simulink model "sampleModel1395_1_sub_sub_sub"  (R2023a)
settings: Solver=VariableStepAuto  StartTime=0.0  StopTime=10.0  RelTol=1e-3
libraries: simulink x1, hdlsllib x1
settings Model: Creator=user1  LastModifiedBy=user1

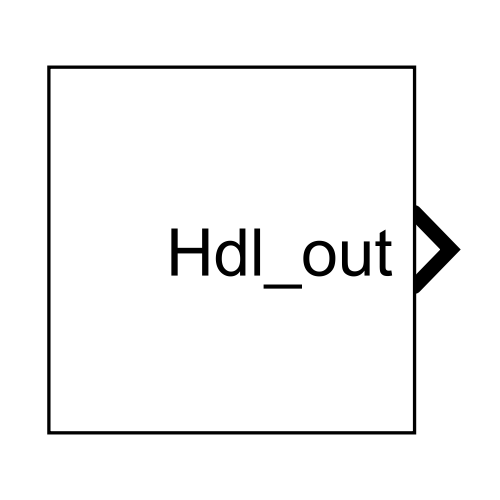
[thumbnail: Simulink's stored preview of the top-level diagram]
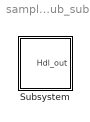
== system sampleModel1395_1_sub_sub_sub ==
  Subsystem : Subsystem

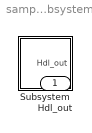
== system sampleModel1395_1_sub_sub_sub/Subsystem ==
  Subsystem : Subsystem
  Hdl_out : Outport  OutDataTypeStr=uint8

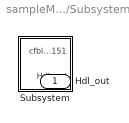
== system sampleModel1395_1_sub_sub_sub/Subsystem/Subsystem ==
  Subsystem : Subsystem
  Hdl_out : Outport  OutDataTypeStr=uint8

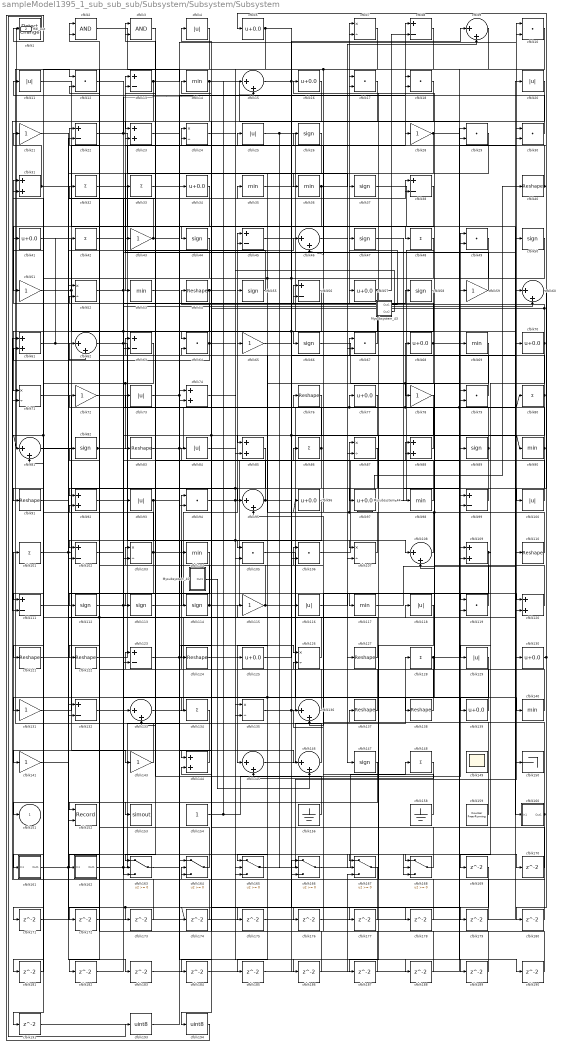
== system sampleModel1395_1_sub_sub_sub/Subsystem/Subsystem/Subsystem ==
  Mysubsystem_40 : Subsystem  TreatAsAtomicUnit=on  RTWFcnName=Mysubsystem_40
      settings: RTWFcnNameOpts=User specified  RTWFileNameOpts=Use function name
  Mysubsystem_43 : Subsystem  TreatAsAtomicUnit=on  RTWFcnName=Mysubsystem_43
      settings: RTWFcnNameOpts=User specified  RTWFileNameOpts=Use function name
  Mysubsystem_44 : Subsystem  TreatAsAtomicUnit=on  RTWFcnName=Mysubsystem_44
      settings: RTWFcnNameOpts=User specified  RTWFileNameOpts=Use function name
  cfblk1 : simulink/Logic and Bit Operations/Detect Change  vinit=0  OutDataTypeStr=uint8
      settings: LibrarySourceBlock=|
      | hdlsllib/Logic and Bit
      | Operations/Detect
      | Change
  cfblk{10,12,17..18,29..30,49,64,67,79,94,105..106,119} (14 alike) : DotProduct  OutDataTypeStr=uint8
  cfblk{4,11,20,25,73,84,93,100,116,118,129} (11 alike) : Abs  OutDataTypeStr=uint8  SaturateOnIntegerOverflow=off
  cfblk{32..33,42,48,80,86,101,128,134,148} (10 alike) : Sum  Inputs=+  OutDataTypeStr=uint8
  cfblk{8,13,22,38,45,56,63,99,102,111,123,132} (12 alike) : Sum  Inputs=+-  OutDataTypeStr=uint8
  cfblk{7,24,52,71,87,103,107,126,135} (9 alike) : Product  Inputs=*/  OutDataTypeStr=uint8  RndMeth=Zero  SaturateOnIntegerOverflow=on
  cfblk{14,35..36,53,69,90,98,104,117,140} (10 alike) : MinMax  OutDataTypeStr=uint8
  cfblk{9,15,46,60,62,81,95,108,133,136,145..146} (12 alike) : Sum  Inputs=|++  OutDataTypeStr=uint8
  cfblk{23,31,61,74,85,88,92,109,120,144} (10 alike) : Sum  OutDataTypeStr=uint8
  cfblk{40,54,76,83,91,110,121..122,124,127,137..138} (12 alike) : Reshape
  cfblk{26,37,44,47,50,55,58,66,82,89,112..114,147} (14 alike) : Signum
  cfblk{21,28,43,51,59,65,72,78,115,131,141,143} (12 alike) : Gain  OutDataTypeStr=uint8
  cfblk{5,16,34,41,57,68,70,77,96..97,125,130,139} (13 alike) : Bias  Bias=0.0  SaturateOnIntegerOverflow=off
  cfblk149 : Scope
      settings: Floating=on
  cfblk150 : Terminator
  cfblk152 : Record  FileSettingsInternal="{\"entries\":[{\"content\":{\"excelSettings\":{\"content\":{},\"type\":\"Streamout.ExcelSettings\"}},\"type\":\"Streamout.FileSettingStorage\",\"uuid\":\"\"}],\"packageUris\":[\"http:\\/\\/schema.mathworks.com\\/mf0\\/streamout_blocks\\/R2020a\"],\"version\":\"1.0\"}"  Layout=[1 1]  SignalsInternal="{\"entries\":[{\"content\":{\"signals\":[{\"content\":{\"blockPath\":[],\"dimensions\":[1],\"domain\":\"\",\"lineColor\":\"#a2142f\",\"plots\":[1],\"port\":1,\"signalID\":10034,\"signalName\":\"cfblk128\"},\"type\":\"RecordBlkView.Signal\",\"uuid\":\"\"},{\"content\":{\"blockPath\":[],\"dimensions\":[1],\"domain\":\"\",\"lineColor\":\"#139fff\",\"plots\":[1],\"port\":2,\"signalID\":10037,\"signalName\":\"cfblk26\"},\"type\":\"RecordBlkView.Signal\",\"uuid\":\"\"}]},\"type\":\"RecordBlkView.InputSignals\",\"uuid\":\"\"}],\"packageUris\":[\"http:\\/\\/schema.mathworks.com\\/mf0\\/streamout_blocks\\/R2020a\"],\"version\":\"1.0\"}"  VisualizationBindings="{\"xyplotplugin\":{\"info\":[{\"series\":[{\"bindingParametersList\":[{\"parameter\":\"X-Axis\",\"signalID\":10034,\"signalName\":\"cfblk128\"},{\"parameter\":\"Y-Axis\",\"signalID\":10037,\"signalName\":\"cfblk26\"}],\"seriesID\":30832}],\"subplotID\":1}]}}"  CompatibilityTag=XY  st=-1
  cfblk153 : ToWorkspace  VariableName=simout  SaveFormat=Timeseries  SampleTime=-1
  cfblk154 : Constant  OutDataTypeStr=uint8  SampleTime=-1
  cfblk156 : Ground
  cfblk158 : Ground
  cfblk159 : hdlsllib/Sources/Counter Free-Running  NumBits=16  tsamp=-1
  cfblk160 : Subsystem
      settings: LibrarySourceBlock=|
      | hdlsllib/Ports &
      | Subsystems/Subsystem
  cfblk161 : Subsystem
      settings: LibrarySourceBlock=|
      | hdlsllib/Ports &
      | Subsystems/Subsystem
  cfblk162 : Subsystem
      settings: LibrarySourceBlock=|
      | hdlsllib/Ports &
      | Subsystems/Subsystem
  cfblk{163..168} (6 alike) : Switch  OutDataTypeStr=uint8  SaturateOnIntegerOverflow=off  InputSameDT=off
  cfblk{169..191} (23 alike) : Delay  SampleTime=1
  cfblk193 : DataTypeConversion  OutDataTypeStr=uint8  SaturateOnIntegerOverflow=off  RndMeth=Floor
  cfblk194 : DataTypeConversion  OutDataTypeStr=uint8  SaturateOnIntegerOverflow=off  RndMeth=Floor
  cfblk2 : Logic  AllPortsSameDT=off  OutDataTypeStr=boolean
  cfblk3 : Logic  AllPortsSameDT=off  OutDataTypeStr=boolean
  cfblk151 : Outport  OutDataTypeStr=uint8  VectorParamsAs1DForOutWhenUnconnected=off
  Hdl_out : Outport  Port=2  OutDataTypeStr=uint8
  wires:
  cfblk92/1 -> cfblk108/1
  cfblk154/1 -> cfblk15/1, cfblk49/1
  cfblk165/1 -> cfblk10/1
  cfblk11/1 -> cfblk48/1
  cfblk112/1 -> cfblk88/2, cfblk117/1
  cfblk97/1 -> cfblk16/1
  cfblk143/1 -> cfblk12/1
  cfblk79/1 -> cfblk22/1
  cfblk122/1 -> cfblk58/1
  cfblk131/1 -> cfblk8/1
  cfblk36/1 -> cfblk175/1, cfblk9/2
  cfblk136/1 -> cfblk94/1
  cfblk70/1 -> cfblk129/1, cfblk4/1, cfblk54/1
  cfblk114/1 -> cfblk82/1, cfblk88/1
  cfblk72/1 -> cfblk25/1
  cfblk15/1 -> cfblk7/2, cfblk67/2, cfblk168/3, cfblk90/1
  cfblk28/1 -> cfblk190/1, cfblk53/1
  cfblk113/1 -> cfblk45/1
  cfblk160/1(Out1) -> cfblk95/2, cfblk101/1
  cfblk162/1(Out1) -> cfblk50/1, cfblk74/1
  cfblk41/1 -> cfblk160/1(In1)
  cfblk101/1 -> cfblk45/2, cfblk143/1
  cfblk106/1 -> cfblk89/1
  cfblk9/1 -> cfblk112/1
  cfblk108/1 -> cfblk73/1, cfblk87/1
  cfblk46/1 -> cfblk87/2
  cfblk64/1 -> cfblk167/2, cfblk61/2, cfblk13/1
  cfblk145/1 -> cfblk128/1
  cfblk121/1 -> cfblk62/2
  cfblk8/1 -> cfblk111/1
  cfblk83/1 -> cfblk38/1, cfblk76/1
  cfblk105/1 -> cfblk140/1
  cfblk159/1 -> cfblk103/1
  cfblk124/1 -> cfblk145/1
  cfblk2/1 -> cfblk74/2
  cfblk62/1 -> cfblk57/1, cfblk114/1
  cfblk57/1 -> cfblk8/2, cfblk163/3, cfblk131/1
  cfblk123/1 -> cfblk188/1, cfblk118/1
  cfblk135/1 -> cfblk179/1, cfblk59/1
  cfblk55/1 -> cfblk13/2
  cfblk73/1 -> cfblk189/1, cfblk18/2
  cfblk24/1 -> cfblk66/1
  cfblk100/1 -> cfblk28/1
  cfblk146/1 -> cfblk12/2
  cfblk37/1 -> cfblk150/1
  cfblk89/1 -> cfblk105/2, cfblk2/2, cfblk68/1
  cfblk12/1 -> cfblk139/1
  cfblk71/1 -> cfblk147/1
  cfblk35/1 -> cfblk98/1
  cfblk95/1 -> cfblk38/2, cfblk84/1
  cfblk51/1 -> cfblk93/1, cfblk24/1
  cfblk52/1 -> cfblk46/1, cfblk64/1
  cfblk68/1 -> cfblk120/2, cfblk31/1, cfblk105/1, cfblk78/1
  cfblk67/1 -> cfblk7/1
  cfblk156/1 -> cfblk63/1
  cfblk109/1 -> cfblk169/1, cfblk136/2
  cfblk31/1 -> cfblk120/1, cfblk21/1
  cfblk119/1 -> cfblk56/2, cfblk96/1
  cfblk7/1 -> cfblk46/2, cfblk153/1
  cfblk86/1 -> cfblk23/2, cfblk113/1
  cfblk4/1 -> cfblk122/1
  cfblk18/1 -> cfblk63/2
  cfblk77/1 -> cfblk85/1
  cfblk90/1 -> cfblk108/2, cfblk65/1, cfblk77/1
  cfblk80/1 -> cfblk97/1, cfblk69/1
  cfblk69/1 -> cfblk138/1
  cfblk17/1 -> cfblk44/1
  cfblk50/1 -> cfblk166/3, cfblk102/1
  cfblk34/1 -> cfblk51/1
  cfblk44/1 -> cfblk161/1(In1)
  cfblk120/1 -> cfblk67/1
  cfblk48/1 -> cfblk181/1, cfblk165/1
  cfblk115/1 -> cfblk9/1, cfblk14/1
  cfblk59/1 -> cfblk43/1
  cfblk144/1 -> cfblk141/1
  cfblk58/1 -> cfblk71/1
  cfblk161/1(Out1) -> cfblk176/1, cfblk167/1
  cfblk29/1 -> cfblk125/1
  cfblk133/1 -> cfblk20/1
  cfblk22/1 -> cfblk170/1, cfblk15/2, cfblk107/2
  cfblk43/1 -> cfblk178/1, cfblk2/1
  cfblk10/1 -> cfblk49/2
  cfblk16/1 -> cfblk111/2
  cfblk49/1 -> cfblk102/2
  cfblk102/1 -> cfblk37/1
  cfblk13/1 -> cfblk71/2, cfblk10/2
  cfblk78/1 -> cfblk163/2, cfblk124/1
  cfblk163/1 -> cfblk55/1
  cfblk63/1 -> cfblk83/1, cfblk91/1
  cfblk76/1 -> cfblk163/1
  cfblk85/1 -> cfblk134/1
  cfblk99/1 -> cfblk92/1
  cfblk81/1 -> cfblk135/1
  cfblk3/1 -> cfblk23/1
  cfblk65/1 -> cfblk168/1
  cfblk53/1 -> cfblk126/1
  cfblk66/1 -> cfblk109/1
  cfblk98/1 -> cfblk3/1
  cfblk32/1 -> cfblk104/1
  cfblk54/1 -> cfblk168/2, cfblk133/2
  cfblk14/1 -> cfblk99/1, cfblk81/1, cfblk151/1
  cfblk158/1 -> cfblk115/1
  cfblk61/1 -> cfblk42/1, cfblk174/1, cfblk173/1
  cfblk94/1 -> cfblk106/2, cfblk29/2
  cfblk148/1 -> cfblk145/2
  cfblk5/1 -> cfblk165/2, cfblk116/1
  cfblk164/1 -> cfblk92/2
  cfblk166/1 -> cfblk148/1
  cfblk23/1 -> cfblk146/1
  cfblk132/1 -> cfblk79/2
  cfblk82/1 -> Hdl_out/1, cfblk107/1
  cfblk25/1 -> cfblk166/2, cfblk130/1
  cfblk128/1 -> cfblk80/1, cfblk30/1, cfblk185/1, cfblk152/1
  cfblk125/1 -> cfblk70/1
  cfblk42/1 -> cfblk60/2
  cfblk40/1 -> cfblk3/2, cfblk5/1
  cfblk60/1 -> cfblk100/1
  cfblk26/1 -> cfblk152/2
  cfblk168/1 -> cfblk137/1
  cfblk117/1 -> cfblk110/1
  cfblk139/1 -> cfblk18/1
  cfblk111/1 -> cfblk35/1
  cfblk30/1 -> cfblk11/1
  cfblk138/1 -> cfblk32/1
  cfblk140/1 -> cfblk123/1
  cfblk127/1 -> cfblk81/2, cfblk72/1
  cfblk45/1 -> cfblk127/1
  cfblk21/1 -> cfblk52/1
  cfblk167/1 -> cfblk164/2
  cfblk137/1 -> cfblk106/1
  cfblk116/1 -> cfblk119/1
  cfblk47/1 -> cfblk99/2
  cfblk88/1 -> cfblk17/1
  cfblk126/1 -> cfblk33/1
  cfblk130/1 -> cfblk180/1, cfblk30/2
  cfblk56/1 -> cfblk121/1
  cfblk87/1 -> cfblk103/2, cfblk135/2
  cfblk93/1 -> cfblk95/1, cfblk162/1(In1)
  cfblk20/1 -> cfblk144/1
  cfblk110/1 -> cfblk56/1
  cfblk33/1 -> cfblk36/1
  cfblk107/1 -> cfblk26/1
  cfblk96/1 -> cfblk165/3, cfblk132/2
  cfblk103/1 -> cfblk123/2, cfblk41/1, cfblk86/1
  cfblk141/1 -> cfblk119/2
  cfblk170/1 -> cfblk24/2
  cfblk134/1 -> cfblk171/1
  cfblk171/1 -> cfblk22/2
  cfblk147/1 -> cfblk172/1
  cfblk172/1 -> cfblk29/1
  cfblk173/1 -> cfblk132/1
  cfblk174/1 -> cfblk52/2
  cfblk175/1 -> cfblk79/1
  cfblk176/1 -> cfblk60/1
  cfblk74/1 -> cfblk177/1
  cfblk177/1 -> cfblk126/2
  cfblk178/1 -> cfblk17/2
  cfblk179/1 -> cfblk61/1
  cfblk180/1 -> cfblk164/3
  cfblk181/1 -> cfblk31/2
  cfblk104/1 -> cfblk182/1
  cfblk182/1 -> cfblk133/1
  cfblk91/1 -> cfblk183/1
  cfblk183/1 -> cfblk166/1
  cfblk38/1 -> cfblk184/1
  cfblk184/1 -> cfblk109/2
  cfblk185/1 -> cfblk167/3
  cfblk84/1 -> cfblk186/1
  cfblk186/1 -> cfblk64/2
  cfblk118/1 -> cfblk187/1
  cfblk187/1 -> cfblk62/1
  cfblk188/1 -> cfblk144/2
  cfblk189/1 -> cfblk164/1
  cfblk190/1 -> cfblk136/1
  cfblk129/1 -> cfblk191/1
  cfblk191/1 -> cfblk94/2
  cfblk1/1 -> cfblk193/1
  cfblk193/1 -> cfblk34/1
  cfblk169/1 -> cfblk194/1
  cfblk194/1 -> cfblk1/1
  Mysubsystem_40/1(Out1) -> cfblk146/2
  Mysubsystem_43/1(Out1) -> cfblk47/1
  Mysubsystem_43/2(Out2) -> cfblk85/2
  Mysubsystem_44/1(Out1) -> cfblk40/1

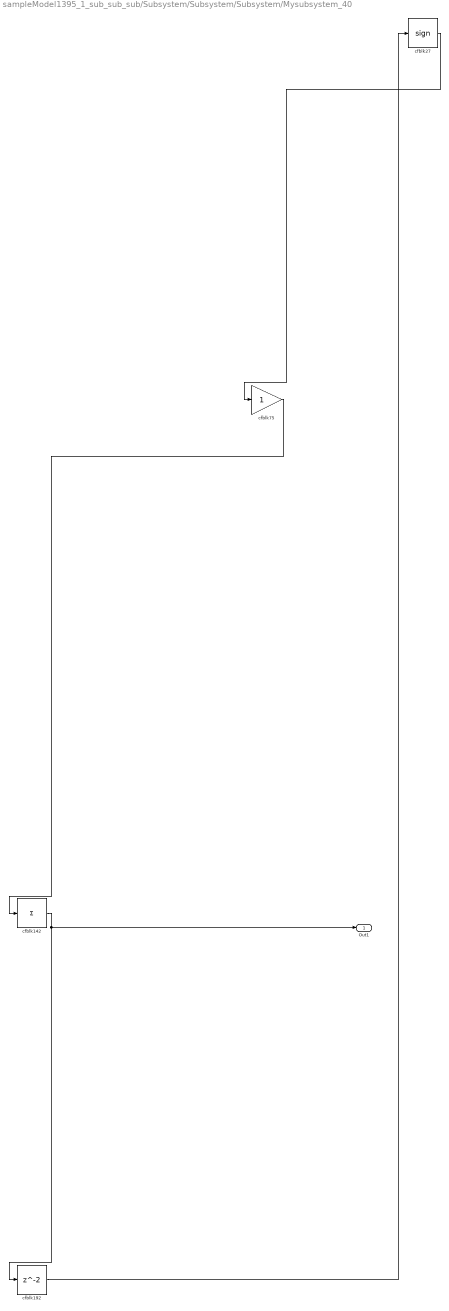
== system sampleModel1395_1_sub_sub_sub/Subsystem/Subsystem/Subsystem/Mysubsystem_40 ==
  cfblk142 : Sum  Inputs=+
  cfblk192 : Delay  SampleTime=1
  cfblk27 : Signum
  cfblk75 : Gain
  Out1 : Outport
  wires:
  cfblk75/1 -> cfblk142/1
  cfblk192/1 -> cfblk27/1
  cfblk142/1 -> cfblk192/1, Out1/1
  cfblk27/1 -> cfblk75/1

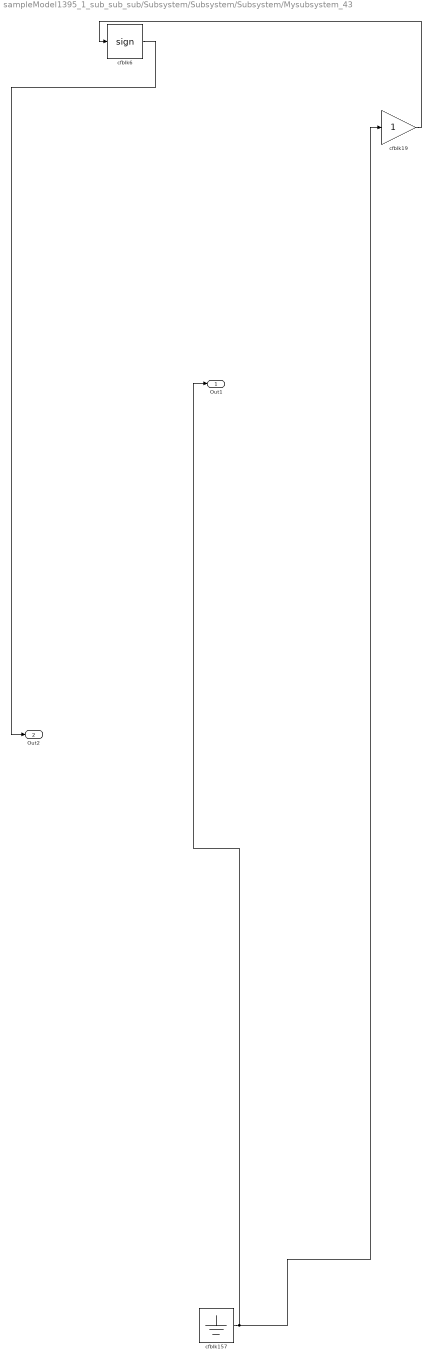
== system sampleModel1395_1_sub_sub_sub/Subsystem/Subsystem/Subsystem/Mysubsystem_43 ==
  cfblk157 : Ground
  cfblk19 : Gain
  cfblk6 : Signum
  Out1 : Outport
  Out2 : Outport  Port=2
  wires:
  cfblk19/1 -> cfblk6/1
  cfblk6/1 -> Out2/1
  cfblk157/1 -> cfblk19/1, Out1/1

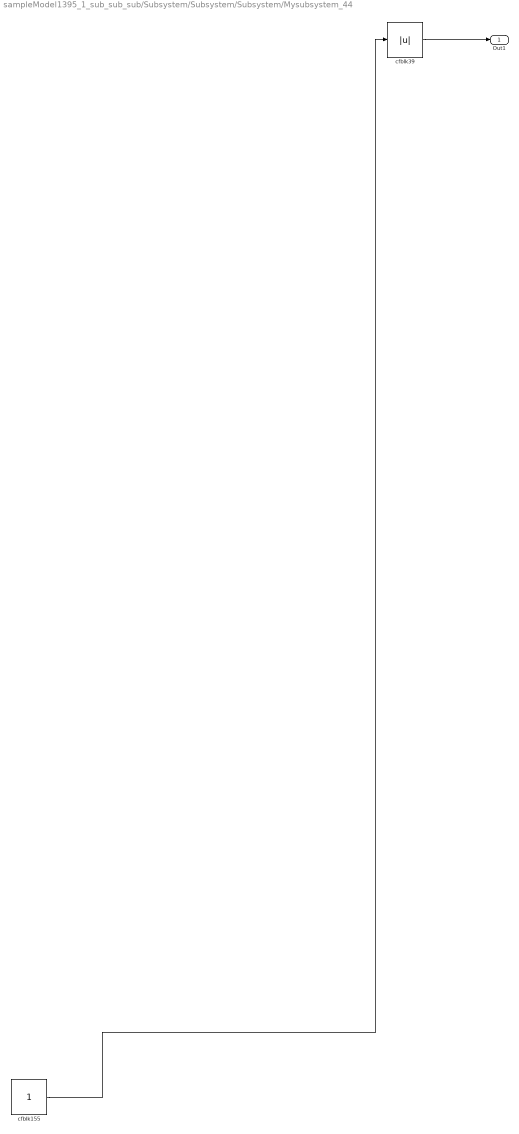
== system sampleModel1395_1_sub_sub_sub/Subsystem/Subsystem/Subsystem/Mysubsystem_44 ==
  cfblk155 : Constant  SampleTime=-1
  cfblk39 : Abs  SaturateOnIntegerOverflow=off
  Out1 : Outport
  wires:
  cfblk39/1 -> Out1/1
  cfblk155/1 -> cfblk39/1

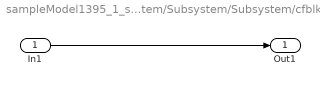
== system sampleModel1395_1_sub_sub_sub/Subsystem/Subsystem/Subsystem/cfblk160 ==
  In1 : Inport
  Out1 : Outport
  wires:
  In1/1 -> Out1/1

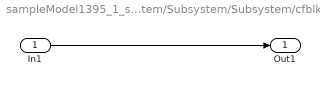
== system sampleModel1395_1_sub_sub_sub/Subsystem/Subsystem/Subsystem/cfblk161 ==
  In1 : Inport
  Out1 : Outport
  wires:
  In1/1 -> Out1/1

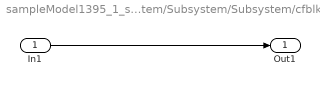
== system sampleModel1395_1_sub_sub_sub/Subsystem/Subsystem/Subsystem/cfblk162 ==
  In1 : Inport
  Out1 : Outport
  wires:
  In1/1 -> Out1/1
